simulink model "example"  (R2020b)
settings: Solver=VariableStepAuto  StartTime=0.0  StopTime=10.0  RelTol=1e-3
settings Model: Creator=apple  LastModifiedBy=apple

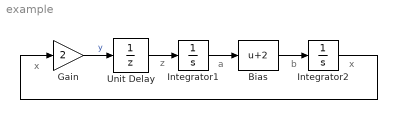
== system example ==
  note: z
  note: x
  note: x
  note: a
  note: b
  "Bias " : Bias  Bias=2
  "Gain " : Gain  Gain=2  SampleTime=1
  "Integrator1 " : Integrator
  "Integrator2 " : Integrator
  "Unit Delay " : UnitDelay  SampleTime=-1  HasFrameUpgradeWarning=on
  wires:
  "Gain "/1 -> "Unit Delay "/1  "y"
  "Integrator1 "/1 -> "Bias "/1
  "Integrator2 "/1 -> "Gain "/1
  "Bias "/1 -> "Integrator2 "/1
  "Unit Delay "/1 -> "Integrator1 "/1
